simulink model "solar_panel_simu"  (R2021a)
settings: Solver=FixedStepAuto  StartTime=0.0  StopTime=10.0  RelTol=1e-3  EnableMultiTasking=on
libraries: arduinolib x9
settings Model: SILPILModeSetting=veronly  ExtModeTrigDuration=2  Creator=AHMED  LastModifiedBy=AHMED
settings OptimizationCC: EnhancedBackFolding=on  PassReuseOutputArgsAs=Individual arguments  ZeroExternalMemoryAtStartup=off  ZeroInternalMemoryAtStartup=off  MaxStackSize=64  OptimizeBlockOrder=speed  DifferentSizesBufferReuse=on  OptimizationCustomize=off  EfficientTunableParamExpr=on
settings DebuggingCC: ParameterTunabilityLossMsg=error
settings HardwareCC: ProdBitPerInt=16  ProdBitPerPointer=16  ProdBitPerSizeT=16  ProdBitPerPtrDiffT=16  ProdLargestAtomicFloat=None  ProdWordSize=8  ProdHWDeviceType=Atmel->AVR
settings SFSimCC: MATLABDynamicMemAlloc=off
settings RTWCC: SystemTargetFile=ert.tlc  HardwareBoard=Arduino Uno  TemplateMakefile=ert_default_tmf  Toolchain=Arduino AVR  BuildConfiguration=Faster Runs
settings CodeAppCC: ForceParamTrailComments=on  IgnoreCustomStorageClasses=off  OperatorAnnotations=on  SimulinkDataObjDesc=on  SFDataObjDesc=on  InsertBlockDesc=on
settings ERTTargetCC: SupportContinuousTime=on  SupportVariableSizeSignals=on  ExtModeStaticAllocSize=250

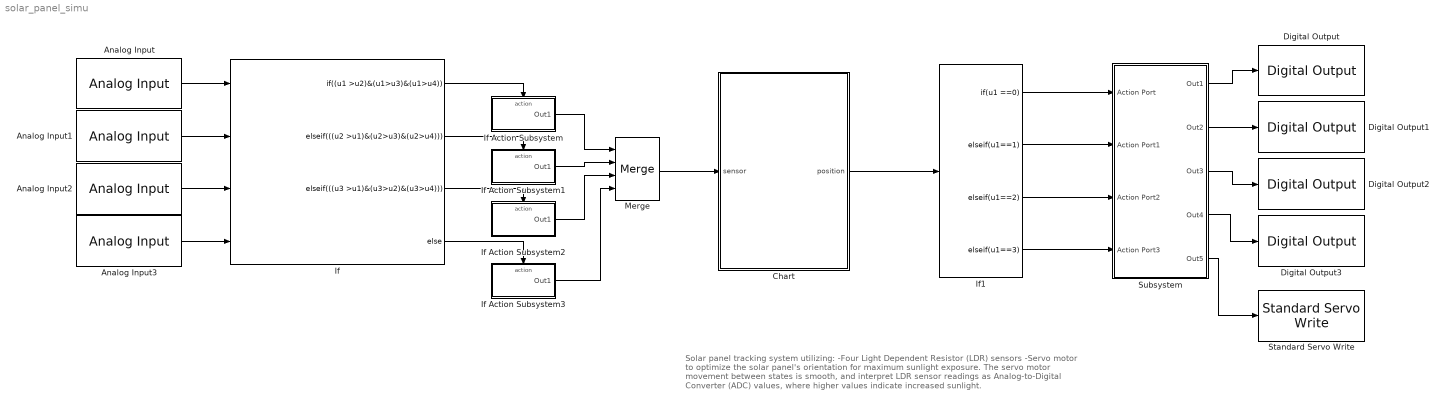
== system solar_panel_simu ==
  note: Solar panel tracking system utilizing:
      | -Four Light Dependent Resistor (LDR) sensors
      | -Servo motor to optimize the solar panel's orientation for maximum sunlight exposure.
      |
      | The servo motor movement between states is smooth, and interpret LDR sensor readings as Analog-to-Digital Converter (ADC) values, where higher values indicate increased sunlight.
  Analog Input : arduinolib/Analog Input  pinNumber=0  ReadResultsOnly=off  ConversionTriggerSource=Software  ExternalTriggerType=uint32( 0 )  OutputDataType=uint16  EnableConversionCompleteNotify=off  EnableOuputStatus=off  SampleTime=-1  blockPlatform=arduino
  Analog Input1 : arduinolib/Analog Input  pinNumber=1  ReadResultsOnly=off  ConversionTriggerSource=Software  ExternalTriggerType=uint32( 0 )  OutputDataType=uint16  EnableConversionCompleteNotify=off  EnableOuputStatus=off  SampleTime=-1  blockPlatform=arduino
  Analog Input2 : arduinolib/Analog Input  pinNumber=2  ReadResultsOnly=off  ConversionTriggerSource=Software  ExternalTriggerType=uint32( 0 )  OutputDataType=uint16  EnableConversionCompleteNotify=off  EnableOuputStatus=off  SampleTime=-1  blockPlatform=arduino
  Analog Input3 : arduinolib/Analog Input  pinNumber=3  ReadResultsOnly=off  ConversionTriggerSource=Software  ExternalTriggerType=uint32( 0 )  OutputDataType=uint16  EnableConversionCompleteNotify=off  EnableOuputStatus=off  SampleTime=-1  blockPlatform=arduino
  Chart : Stateflow chart  TreatAsAtomicUnit=on
  Digital Output : arduinolib/Digital Output  pinNumber=13  Direction=output  blockPlatform=arduino
  Digital Output1 : arduinolib/Digital Output  pinNumber=12  Direction=output  blockPlatform=arduino
  Digital Output2 : arduinolib/Digital Output  pinNumber=11  Direction=output  blockPlatform=arduino
  Digital Output3 : arduinolib/Digital Output  pinNumber=10  Direction=output  blockPlatform=arduino
  If : If  NumInputs=4  IfExpression=(u1 >u2)&(u1>u3)&(u1>u4)  ElseIfExpressions=((u2 >u1)&(u2>u3)&(u2>u4)),((u3 >u1)&(u3>u2)&(u3>u4))
  If Action Subsystem : Subsystem  TreatAsAtomicUnit=on
  If Action Subsystem1 : Subsystem  TreatAsAtomicUnit=on
  If Action Subsystem2 : Subsystem  TreatAsAtomicUnit=on
  If Action Subsystem3 : Subsystem  TreatAsAtomicUnit=on
  If1 : If  IfExpression=u1 ==0  ElseIfExpressions=u1==1 , u1==2 , u1==3  ShowElse=off
  Merge : Merge  Inputs=4
  Standard Servo Write : arduinolib/Standard Servo Write  pinNumber=9  ServoIndex=0  blockPlatform=ARDUINO
  Subsystem : Subsystem
  wires:
  Chart/1(position) -> If1/1
  If/1 -> If Action Subsystem/Action
  If/2 -> If Action Subsystem1/Action
  If/3 -> If Action Subsystem2/Action
  If/4 -> If Action Subsystem3/Action
  If Action Subsystem/1(Out1) -> Merge/1
  If Action Subsystem1/1(Out1) -> Merge/2
  If Action Subsystem2/1(Out1) -> Merge/3
  If Action Subsystem3/1(Out1) -> Merge/4
  Merge/1 -> Chart/1(sensor)
  Analog Input/1 -> If/1
  Analog Input3/1 -> If/4
  Analog Input2/1 -> If/3
  Analog Input1/1 -> If/2
  If1/1 -> Subsystem/1(Action Port)
  If1/2 -> Subsystem/2(Action Port1)
  If1/3 -> Subsystem/3(Action Port2)
  If1/4 -> Subsystem/4(Action Port3)
  Subsystem/1(Out1) -> Digital Output/1
  Subsystem/2(Out2) -> Digital Output1/1
  Subsystem/3(Out3) -> Digital Output2/1
  Subsystem/4(Out4) -> Digital Output3/1
  Subsystem/5(Out5) -> Standard Servo Write/1

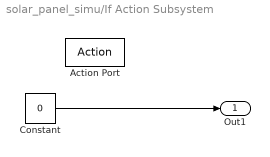
== system solar_panel_simu/If Action Subsystem ==
  Action Port : ActionPort  ActionPortLabel=if((u1 >u2)&(u1>u3)&(u1>u4))
  Constant : Constant  Value=0
  Out1 : Outport
  wires:
  Constant/1 -> Out1/1

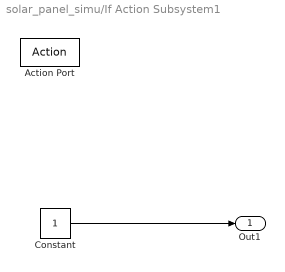
== system solar_panel_simu/If Action Subsystem1 ==
  Action Port : ActionPort  ActionPortLabel=elseif(((u2 >u1)&(u2>u3)&(u2>u4)))
  Constant : Constant
  Out1 : Outport
  wires:
  Constant/1 -> Out1/1

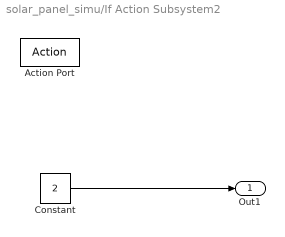
== system solar_panel_simu/If Action Subsystem2 ==
  Action Port : ActionPort  ActionPortLabel=elseif(((u3 >u1)&(u3>u2)&(u3>u4)))
  Constant : Constant  Value=2
  Out1 : Outport
  wires:
  Constant/1 -> Out1/1

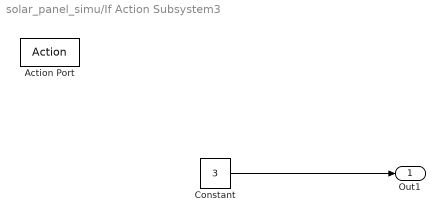
== system solar_panel_simu/If Action Subsystem3 ==
  Action Port : ActionPort  ActionPortLabel=else
  Constant : Constant  Value=3
  Out1 : Outport
  wires:
  Constant/1 -> Out1/1

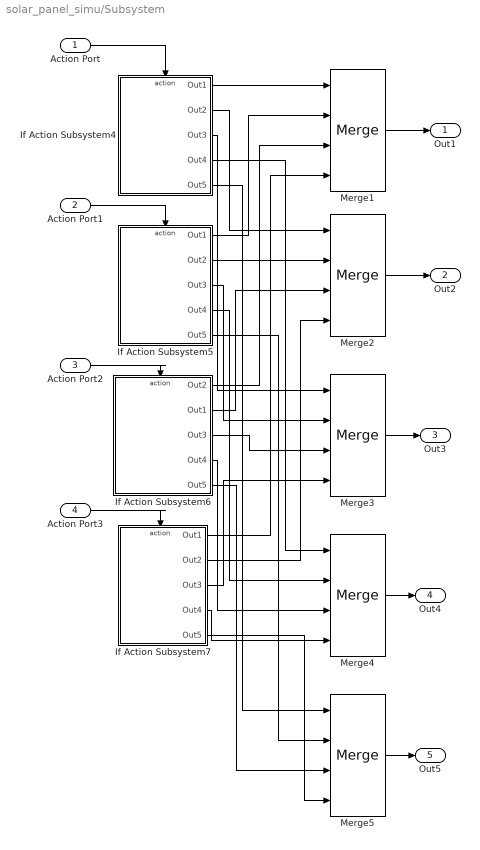
== system solar_panel_simu/Subsystem ==
  Action Port : Inport
  Action Port1 : Inport  Port=2
  Action Port2 : Inport  Port=3
  Action Port3 : Inport  Port=4
  If Action Subsystem4 : Subsystem  TreatAsAtomicUnit=on
  If Action Subsystem5 : Subsystem  TreatAsAtomicUnit=on
  If Action Subsystem6 : Subsystem  TreatAsAtomicUnit=on
  If Action Subsystem7 : Subsystem  TreatAsAtomicUnit=on
  Merge{1..5} (5 alike) : Merge  Inputs=4
  Out1 : Outport
  Out2 : Outport  Port=2
  Out3 : Outport  Port=3
  Out4 : Outport  Port=4
  Out5 : Outport  Port=5
  wires:
  Action Port3/1 -> If Action Subsystem7/Action
  Action Port2/1 -> If Action Subsystem6/Action
  Action Port/1 -> If Action Subsystem4/Action
  Action Port1/1 -> If Action Subsystem5/Action
  If Action Subsystem4/1(Out1) -> Merge1/1
  If Action Subsystem5/1(Out1) -> Merge1/2
  If Action Subsystem6/1(Out2) -> Merge1/3
  If Action Subsystem7/1(Out1) -> Merge1/4
  If Action Subsystem4/2(Out2) -> Merge2/1
  If Action Subsystem5/2(Out2) -> Merge2/2
  If Action Subsystem6/2(Out1) -> Merge2/3
  If Action Subsystem7/2(Out2) -> Merge2/4
  If Action Subsystem7/3(Out3) -> Merge3/4
  If Action Subsystem6/3(Out3) -> Merge3/3
  If Action Subsystem5/3(Out3) -> Merge3/2
  If Action Subsystem4/3(Out3) -> Merge3/1
  If Action Subsystem4/4(Out4) -> Merge4/1
  If Action Subsystem5/4(Out4) -> Merge4/2
  If Action Subsystem6/4(Out4) -> Merge4/3
  If Action Subsystem7/4(Out4) -> Merge4/4
  If Action Subsystem4/5(Out5) -> Merge5/1
  If Action Subsystem5/5(Out5) -> Merge5/2
  If Action Subsystem6/5(Out5) -> Merge5/3
  If Action Subsystem7/5(Out5) -> Merge5/4
  Merge1/1 -> Out1/1
  Merge2/1 -> Out2/1
  Merge3/1 -> Out3/1
  Merge4/1 -> Out4/1
  Merge5/1 -> Out5/1

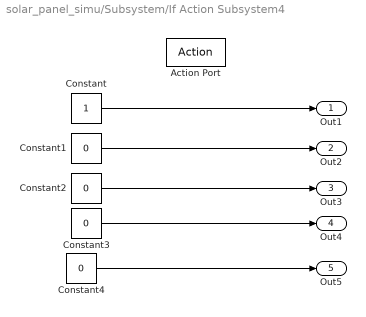
== system solar_panel_simu/Subsystem/If Action Subsystem4 ==
  Action Port : ActionPort  ActionPortLabel=if(u1 ==0)
  Constant : Constant
  Constant{1..4} (4 alike) : Constant  Value=0
  Out1 : Outport
  Out2 : Outport  Port=2
  Out3 : Outport  Port=3
  Out4 : Outport  Port=4
  Out5 : Outport  Port=5
  wires:
  Constant/1 -> Out1/1
  Constant1/1 -> Out2/1
  Constant2/1 -> Out3/1
  Constant3/1 -> Out4/1
  Constant4/1 -> Out5/1

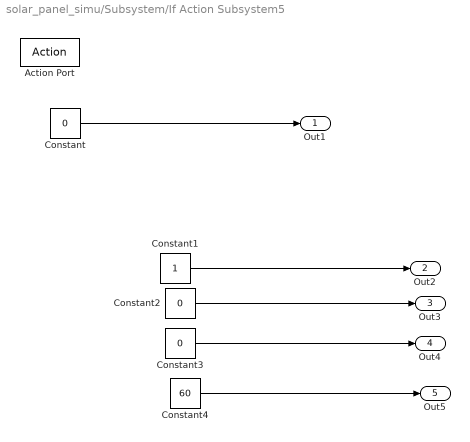
== system solar_panel_simu/Subsystem/If Action Subsystem5 ==
  Action Port : ActionPort  ActionPortLabel=elseif(u1==1 )
  Constant : Constant  Value=0
  Constant1 : Constant
  Constant2 : Constant  Value=0
  Constant3 : Constant  Value=0
  Constant4 : Constant  Value=60
  Out1 : Outport
  Out2 : Outport  Port=2
  Out3 : Outport  Port=3
  Out4 : Outport  Port=4
  Out5 : Outport  Port=5
  wires:
  Constant/1 -> Out1/1
  Constant1/1 -> Out2/1
  Constant2/1 -> Out3/1
  Constant3/1 -> Out4/1
  Constant4/1 -> Out5/1

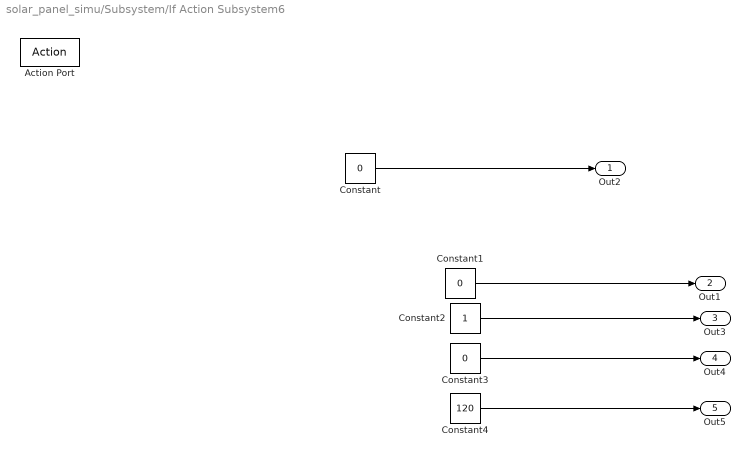
== system solar_panel_simu/Subsystem/If Action Subsystem6 ==
  Action Port : ActionPort  ActionPortLabel=elseif( u1==2 )
  Constant : Constant  Value=0
  Constant1 : Constant  Value=0
  Constant2 : Constant
  Constant3 : Constant  Value=0
  Constant4 : Constant  Value=120
  Out2 : Outport
  Out1 : Outport  Port=2
  Out3 : Outport  Port=3
  Out4 : Outport  Port=4
  Out5 : Outport  Port=5
  wires:
  Constant/1 -> Out2/1
  Constant1/1 -> Out1/1
  Constant2/1 -> Out3/1
  Constant3/1 -> Out4/1
  Constant4/1 -> Out5/1

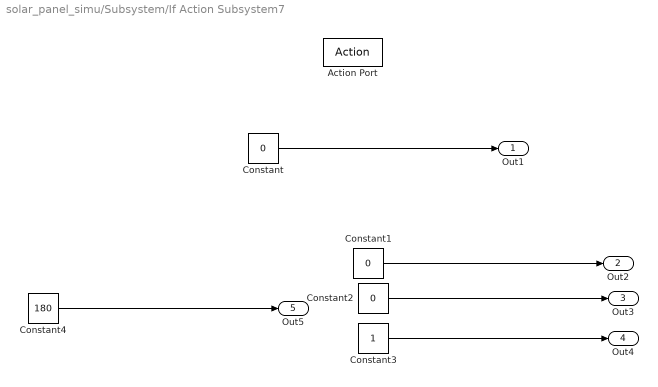
== system solar_panel_simu/Subsystem/If Action Subsystem7 ==
  Action Port : ActionPort  ActionPortLabel=elseif( u1==3)
  Constant : Constant  Value=0
  Constant1 : Constant  Value=0
  Constant2 : Constant  Value=0
  Constant3 : Constant
  Constant4 : Constant  Value=180
  Out1 : Outport
  Out2 : Outport  Port=2
  Out3 : Outport  Port=3
  Out4 : Outport  Port=4
  Out5 : Outport  Port=5
  wires:
  Constant/1 -> Out1/1
  Constant1/1 -> Out2/1
  Constant2/1 -> Out3/1
  Constant3/1 -> Out4/1
  Constant4/1 -> Out5/1

== stateflow chart solar_panel_simu/Chart ==
  state South
    en:
    position=1;
    during:
    position=1;
  state East
    en:
    position=2;
    during:
    position=2;
  state North
    en:
    position=0;
    during:
    position=0;
  state West
    en:
    position=3;
    during:
    position=3;
  (junction 11) -> South [order 4] : [sensor == 1]
  South -> (junction 11) : [sensor ~= 1]
  (junction 6) -> South [order 1] : [sensor == 1]
  (junction 11) -> East [order 2] : [sensor == 2]
  (default) -> North
  East -> (junction 11) : [sensor ~= 2]
  (junction 11) -> North [order 1] : [sensor == 0]
  (junction 11) -> West [order 3] : [sensor== 3]
  West -> (junction 11) : [sensor ~= 3]
  North -> (junction 6) : [sensor ~= 0]
  (junction 6) -> East [order 2] : [sensor == 2]
  (junction 6) -> West [order 3] : [sensor == 3]
  data: sensor input; position output
